simulink model "prodc20Vfinal"  (R2021b)
settings: Solver=VariableStepAuto  StartTime=0.0  StopTime=0.01  RelTol=1e-3
undefined symbols (not defined in the file): magnitude
libraries: dspstat3 x5, commfilt2 x2, commrflib2 x1
settings Model: Creator=Lorenzo Bisulli  LastModifiedBy=utente

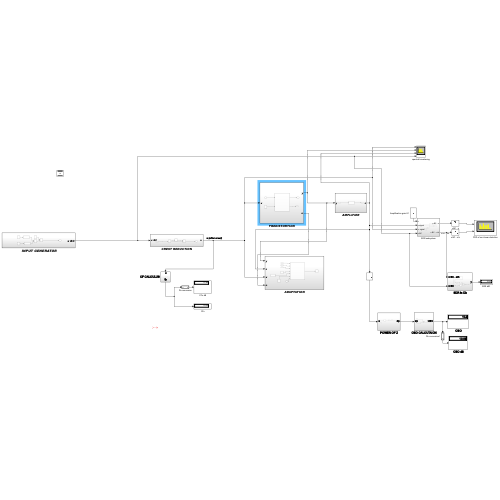
[thumbnail: Simulink's stored preview of the top-level diagram]
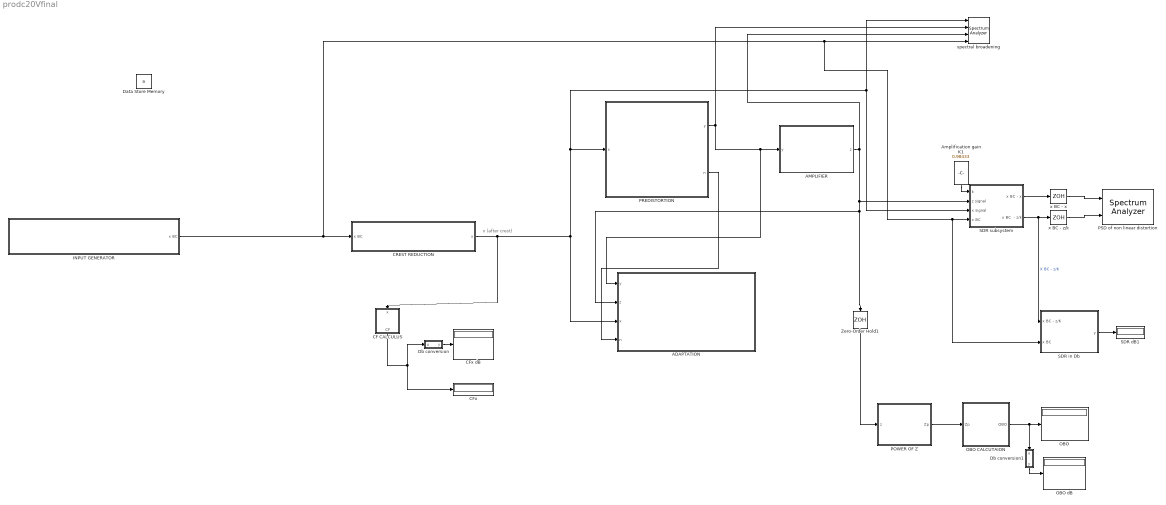
== system prodc20Vfinal ==
  note: x (after crest)
  " CFx" : Display
  " CFx dB" : Display
  " INPUT GENERATOR" : Subsystem
  " OBO" : Display
  " OBO dB" : Display
  ADAPTATION : Subsystem
  AMPLIFIER : Subsystem
  Amplification gain K1 : Constant  Value=0.98433
  CF CALCULUS : Subsystem
  CREST REDUCTION : Subsystem
  Data Store Memory : DataStoreMemory  DataStoreName=a  ReadBeforeWriteMsg=warning  WriteAfterWriteMsg=warning  WriteAfterReadMsg=warning  InitialValue=ones(1,21) + 1i*zeros(1,21)  ShowAdditionalParam=off
      settings: SignalType=complex
  Db conversion : MATLAB Function  TreatAsAtomicUnit=on
  Db conversion1 : MATLAB Function  TreatAsAtomicUnit=on
  OBO CALCUTAION : Subsystem
  POWER OF Z : Subsystem
  PREDISTORTION : Subsystem
  PSD of non linear distortion : SpectrumAnalyzer  NumInputPorts=2
  SDR dB1 : Display
  SDR in Db : Subsystem
  SDR subsystem : Subsystem
  Zero-Order Hold1 : ZeroOrderHold  SampleTime=-1
  spectral broadening : SpectrumAnalyzer  NumInputPorts=4
  x BC - x : ZeroOrderHold  SampleTime=-1
  x BC - z/k : ZeroOrderHold  SampleTime=-1
  wires:
  " INPUT GENERATOR"/1(x BC) -> SDR in Db/2(x BC), SDR subsystem/4(x BC), spectral broadening/4, CREST REDUCTION/1(x BC)
  PREDISTORTION/1(y) -> spectral broadening/2, ADAPTATION/1(y), AMPLIFIER/1(y)
  AMPLIFIER/1(z) -> spectral broadening/3, SDR subsystem/2(z signal), Zero-Order Hold1/1, ADAPTATION/2(z)
  SDR subsystem/2(x BC  - z/k) -> SDR in Db/1(x BC - z/K), x BC - z/k/1  "X BC - z/K"
  Amplification gain K1/1 -> SDR subsystem/1(k)
  CREST REDUCTION/1("x ") -> CF CALCULUS/1(x), spectral broadening/1, SDR subsystem/3(" x signal"), PREDISTORTION/1(x), ADAPTATION/3(x)
  SDR subsystem/1(x BC - x) -> x BC - x/1
  x BC - x/1 -> PSD of non linear distortion/1
  x BC - z/k/1 -> PSD of non linear distortion/2
  SDR in Db/1(y) -> SDR dB1/1
  CF CALCULUS/1(CF) -> " CFx"/1, Db conversion/1(u)
  Db conversion/1(y) -> " CFx dB"/1
  Zero-Order Hold1/1 -> POWER OF Z/1(z)
  POWER OF Z/1(Zp) -> OBO CALCUTAION/1(Zp)
  OBO CALCUTAION/1(OBO) -> Db conversion1/1(u), " OBO"/1
  Db conversion1/1(y) -> " OBO dB"/1
  ? -> ?
  PREDISTORTION/2(n) -> ADAPTATION/4(n)

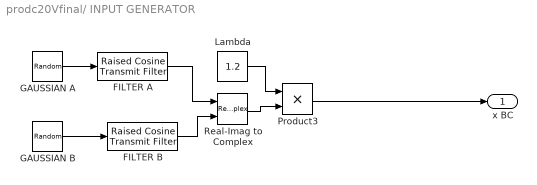
== system prodc20Vfinal/ INPUT GENERATOR ==
  FILTER A : commfilt2/Raised Cosine Transmit Filter  filtType=Square root  R=0.2  filtSpan=80  N=8  filterGain=1  RateOptions=Allow multirate processing  framing=Mute  checkCoeff=off  variableName=rcTxFilt  checkGain=Normalized  sampMode=Mute  saveAsFlag=0  currentFiltSpan=80  D=(80)/2  launchFVT=on  roundingMode=Floor  overflowMode=off  coeffDataTypeStr=Inherit: Same word length as input  coeffMin=[]  coeffMax=[]  coeffLastDataTypeStr=Inherit: Same word length as input  outputDataTypeStr=Inherit: Same as accumulator  outputMin=[]  outputMax=[]  outputLastDataTypeStr=Inherit: Same as accumulator
  FILTER B : commfilt2/Raised Cosine Transmit Filter  filtType=Square root  R=0.2  filtSpan=80  N=8  filterGain=1  RateOptions=Allow multirate processing  framing=Mute  checkCoeff=off  variableName=rcTxFilt1  checkGain=Normalized  sampMode=Mute  saveAsFlag=0  currentFiltSpan=80  D=(80)/2  launchFVT=on  roundingMode=Floor  overflowMode=off  coeffDataTypeStr=Inherit: Same word length as input  coeffMin=[]  coeffMax=[]  coeffLastDataTypeStr=Inherit: Same word length as input  outputDataTypeStr=Inherit: Same as accumulator  outputMin=[]  outputMax=[]  outputLastDataTypeStr=Inherit: Same as accumulator
  GAUSSIAN A : RandomNumber  Variance=0.5  Seed=1  SampleTime=2e-7
  GAUSSIAN B : RandomNumber  Variance=0.5  Seed=2  SampleTime=2e-7
  Lambda : Constant  Value=1.2
  Product3 : Product
  Real-Imag to Complex : RealImagToComplex
  x BC : Outport
  wires:
  Product3/1 -> x BC/1
  GAUSSIAN A/1 -> FILTER A/1
  FILTER A/1 -> Real-Imag to Complex/1
  GAUSSIAN B/1 -> FILTER B/1
  Lambda/1 -> Product3/1
  Real-Imag to Complex/1 -> Product3/2
  FILTER B/1 -> Real-Imag to Complex/2

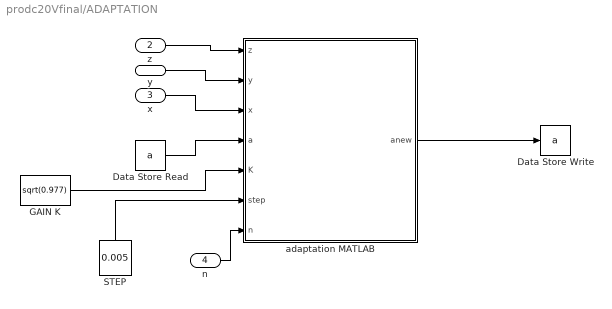
== system prodc20Vfinal/ADAPTATION ==
  y : Inport
  z : Inport  Port=2
  x : Inport  Port=3
  n : Inport  Port=4
  Data Store Read : DataStoreRead  DataStoreName=a  IndexOptions=Index vector (dialog)  Indices=1  OutputSizes=1
  Data Store Write : DataStoreWrite  DataStoreName=a  IndexOptions=Index vector (dialog)  Indices=1  OutputSizes=1
  GAIN K : Constant  Value=sqrt(0.977)
  STEP : Constant  Value=0.005
  adaptation MATLAB : MATLAB Function  TreatAsAtomicUnit=on
  wires:
  y/1 -> adaptation MATLAB/2(y)
  GAIN K/1 -> adaptation MATLAB/5(K)
  x/1 -> adaptation MATLAB/3(x)
  STEP/1 -> adaptation MATLAB/6(step)
  z/1 -> adaptation MATLAB/1(z)
  Data Store Read/1 -> adaptation MATLAB/4(a)
  adaptation MATLAB/1(anew) -> Data Store Write/1
  n/1 -> adaptation MATLAB/7(n)

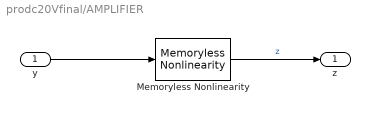
== system prodc20Vfinal/AMPLIFIER ==
  y : Inport
  Memoryless Nonlinearity : commrflib2/Memoryless Nonlinearity  model_select=Rapp model  linGaindB=0  GindB=0  iip3=30  am2pm=10  LPwrLimAMPM=10  UPwrLimAMPM=inf  amam=[2.1587 1.1517]  ampm=[4.0033 9.1040]  x=[8.1081 1.5413 6.5202 -0.0718]  y=[4.6645 2.0965 10.88 -0.003]  p=3  GoutdB=0  vsat=1
      settings: SourceProductBaseCode=CM
  z : Outport
  wires:
  y/1 -> Memoryless Nonlinearity/1
  Memoryless Nonlinearity/1 -> z/1  "z"

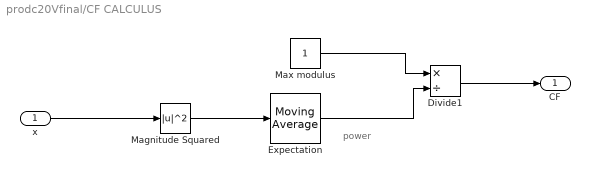
== system prodc20Vfinal/CF CALCULUS ==
  note: power
  x : Inport
  Divide1 : Product  Inputs=*/
  Expectation : dspstat3/Moving Average  Method=Sliding window  ForgettingFactorPort=off  SpecifyWindowLength=on  WindowLength=50000  ForgettingFactor=0.9  SimulateUsing=Code generation
  Magnitude Squared : Math  Operator=magnitude^2  SaturateOnIntegerOverflow=on
  Max modulus : Constant
  CF : Outport
  wires:
  Max modulus/1 -> Divide1/1
  Expectation/1 -> Divide1/2
  x/1 -> Magnitude Squared/1
  Divide1/1 -> CF/1
  Magnitude Squared/1 -> Expectation/1

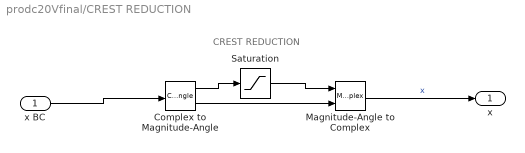
== system prodc20Vfinal/CREST REDUCTION ==
  note: CREST REDUCTION
  x BC : Inport
  Complex to Magnitude-Angle : ComplexToMagnitudeAngle
  Magnitude-Angle to Complex : MagnitudeAngleToComplex
  Saturation : Saturate  UpperLimit=1  LowerLimit=0  LinearizeAsGain=off
  "x " : Outport
  wires:
  Complex to Magnitude-Angle/1 -> Saturation/1
  Complex to Magnitude-Angle/2 -> Magnitude-Angle to Complex/2
  Magnitude-Angle to Complex/1 -> "x "/1  "x"
  x BC/1 -> Complex to Magnitude-Angle/1
  Saturation/1 -> Magnitude-Angle to Complex/1

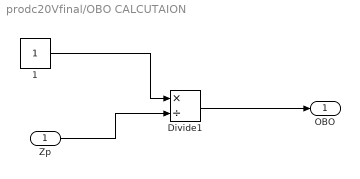
== system prodc20Vfinal/OBO CALCUTAION ==
  Zp : Inport
  1 : Constant
  Divide1 : Product  Inputs=*/
  OBO : Outport
  wires:
  1/1 -> Divide1/1
  Zp/1 -> Divide1/2
  Divide1/1 -> OBO/1

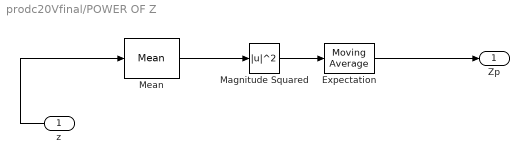
== system prodc20Vfinal/POWER OF Z ==
  z : Inport
  Expectation : dspstat3/Moving Average  Method=Sliding window  ForgettingFactorPort=off  SpecifyWindowLength=on  WindowLength=1500  ForgettingFactor=0.9  SimulateUsing=Code generation
  Magnitude Squared : Math  Operator=magnitude^2  SaturateOnIntegerOverflow=on
  Mean : dspstat3/Mean  run=off  InputProcessing=Columns as channels (frame based)  reset_popup=None  directionMode=Each column  dimension=1  roiEnable=off  roiType=Rectangles  roiPortion=Entire ROI  roiOutput=Individual statistics for each ROI  roiFlag=off  roundingMode=Floor  overflowMode=off  outputDataTypeStr=Inherit: Same as accumulator  outputMin=[]  outputMax=[]  outputLastDataTypeStr=Inherit: Same as accumulator
  Zp : Outport
  wires:
  Magnitude Squared/1 -> Expectation/1
  Expectation/1 -> Zp/1
  Mean/1 -> Magnitude Squared/1
  z/1 -> Mean/1

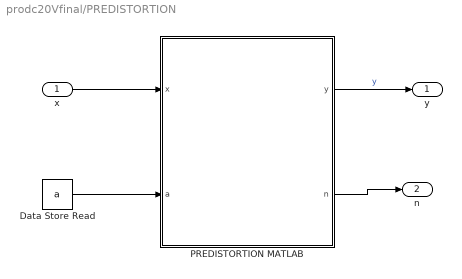
== system prodc20Vfinal/PREDISTORTION ==
  x : Inport
  Data Store Read : DataStoreRead  DataStoreName=a  IndexOptions=Index vector (dialog)  Indices=1  OutputSizes=1
  PREDISTORTION MATLAB : MATLAB Function  TreatAsAtomicUnit=on
  y : Outport
  n : Outport  Port=2
  wires:
  PREDISTORTION MATLAB/1(y) -> y/1  "y"
  x/1 -> PREDISTORTION MATLAB/1(x)
  Data Store Read/1 -> PREDISTORTION MATLAB/2(a)
  PREDISTORTION MATLAB/2(n) -> n/1

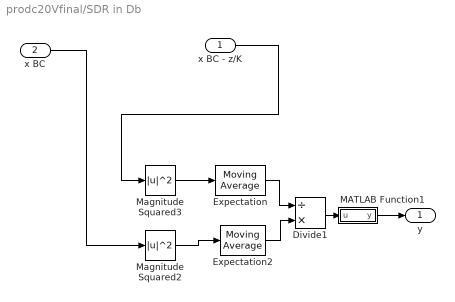
== system prodc20Vfinal/SDR in Db ==
  x BC - z/K : Inport
  x BC : Inport  Port=2
  Divide1 : Product  Inputs=/*
  Expectation : dspstat3/Moving Average  Method=Sliding window  ForgettingFactorPort=off  SpecifyWindowLength=on  WindowLength=1000000  ForgettingFactor=0.9  SimulateUsing=Code generation
  Expectation2 : dspstat3/Moving Average  Method=Sliding window  ForgettingFactorPort=off  SpecifyWindowLength=on  WindowLength=1000000  ForgettingFactor=0.9  SimulateUsing=Code generation
  MATLAB Function1 : MATLAB Function  TreatAsAtomicUnit=on
  Magnitude Squared2 : Math  Operator=magnitude^2  SaturateOnIntegerOverflow=on
  Magnitude Squared3 : Math  Operator=magnitude^2  SaturateOnIntegerOverflow=on
  y : Outport
  wires:
  Magnitude Squared2/1 -> Expectation2/1
  MATLAB Function1/1(y) -> y/1
  x BC - z/K/1 -> Magnitude Squared3/1
  Expectation/1 -> Divide1/1
  Magnitude Squared3/1 -> Expectation/1
  Expectation2/1 -> Divide1/2
  Divide1/1 -> MATLAB Function1/1(u)
  x BC/1 -> Magnitude Squared2/1

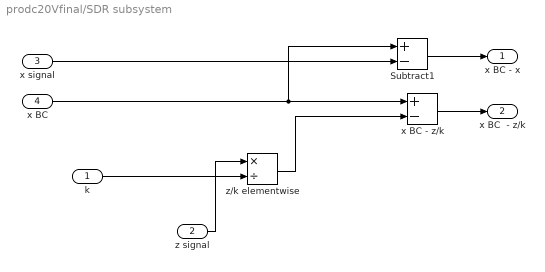
== system prodc20Vfinal/SDR subsystem ==
  k : Inport
  z signal : Inport  Port=2
  " x signal" : Inport  Port=3
  x BC : Inport  Port=4
  "     z/k elementwise" : Product  Inputs=*/
  "    x BC - z/k" : Sum  Inputs=+-
  Subtract1 : Sum  Inputs=+-
  x BC - x : Outport
  x BC  - z/k : Outport  Port=2
  wires:
  "    x BC - z/k"/1 -> x BC  - z/k/1
  "     z/k elementwise"/1 -> "    x BC - z/k"/2
  z signal/1 -> "     z/k elementwise"/1
  x BC/1 -> Subtract1/1, "    x BC - z/k"/1
  " x signal"/1 -> Subtract1/2
  Subtract1/1 -> x BC - x/1
  k/1 -> "     z/k elementwise"/2

== matlab function prodc20Vfinal/PREDISTORTION/PREDISTORTION MATLAB ==
  data: x input; y output; a input; n output
function [y,n] = predistort(x, a)
%N=20 

N = 20;

delta = 1/(2*N);

I = [delta: 2*delta: 1 inf];
%VETTORE CHE VIENE SOVRASCRITTO PER TROVARE LA A 
k = [1 : N+1 ];
k = find(abs(x)<=I);
n=k(1);

P = ((abs(x) -(2*n+1)*delta) * (a(min(n+1,N+1)) -a(n)) / (2*delta)) + ((a(min(n+1,N+1)) *a(n)) /2);


y = complex(P* x);

== matlab function prodc20Vfinal/Db conversion1 ==
  data: u input; y output
function y = lintodb(u)
y = 10.*log10(u);

== matlab function prodc20Vfinal/ADAPTATION/adaptation MATLAB ==
  data: z input; y input; x input; a input; anew output; K input; step input; n input
function anew = adapt(z, y, x, a, K, step,n)
asub = a;
    
    
  
asub(n) = asub(n) - step*(z-K*x)*conj(z)*conj(x)/conj(y);
                %formula from slide 28. The gradient is implemented using a
                %small constant (step) multiplied by k, that increases.
                
anew = asub;
end

== matlab function prodc20Vfinal/SDR in Db/MATLAB Function1 ==
  data: u input; y output
function y = lintodb(u)
y = mean(10.*log10(u));

== matlab function prodc20Vfinal/Db conversion ==
  data: u input; y output
function y = lintodb(u)
y = mean(10.*log10(u));
